simulink model "SD_Model"  (R2023b)
settings: Solver=FixedStepAuto  StartTime=1  StopTime=20  FixedStep=1  RelTol=1e-3
undefined symbols (not defined in the file): DiscIntNeverNeededParam
settings Model: Creator=eddyp  LastModifiedBy=eddyp

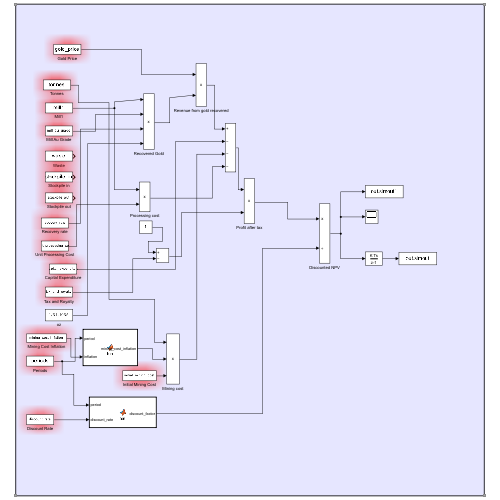
[thumbnail: Simulink's stored preview of the top-level diagram]
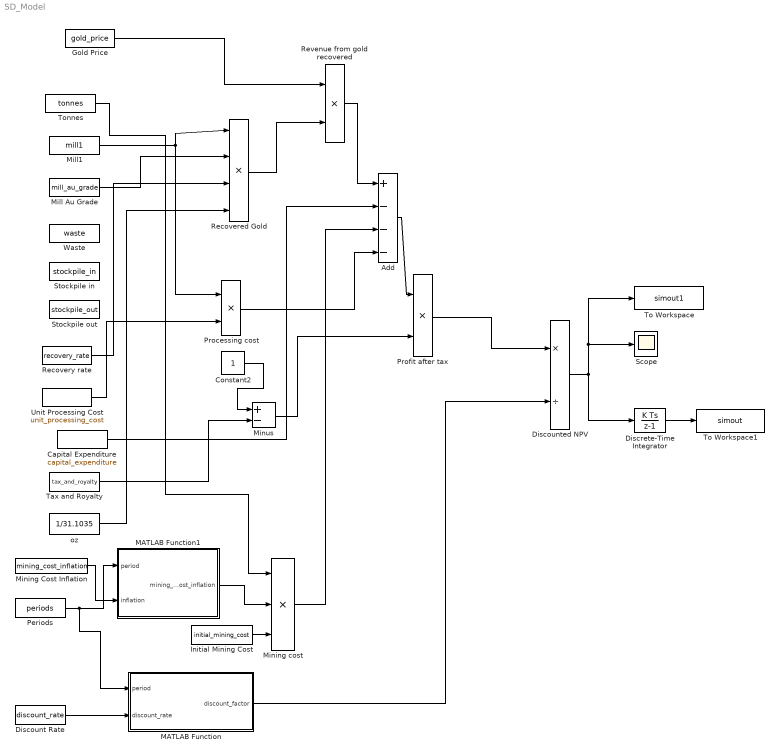
== system SD_Model ==
  Add : Sum  Inputs=+---
  Capital Expenditure : FromWorkspace  VariableName=capital_expenditure
  Constant2 : Constant
  Discount Rate : FromWorkspace  VariableName=discount_rate
  Discounted NPV : Product  Inputs=*/
  Discrete-Time Integrator : DiscreteIntegrator  SampleTime=-1  ICPrevOutput=DiscIntNeverNeededParam  ICPrevScaledInput=DiscIntNeverNeededParam
  Gold Price : FromWorkspace  VariableName=gold_price
  Initial Mining Cost : FromWorkspace  VariableName=initial_mining_cost
  MATLAB Function : MATLAB Function  TreatAsAtomicUnit=on
  MATLAB Function1 : MATLAB Function  TreatAsAtomicUnit=on
  Mill Au Grade : FromWorkspace  VariableName=mill_au_grade
  Mill1 : FromWorkspace  VariableName=mill1
  Mining Cost Inflation : FromWorkspace  VariableName=mining_cost_inflation
  Mining cost : Product  Inputs=3
  Minus : Sum  Inputs=+-
  Periods : FromWorkspace  VariableName=periods
  Processing cost : Product
  Profit after tax : Product
  Recovered Gold : Product  Inputs=4
  Recovery rate : FromWorkspace  VariableName=recovery_rate
  Revenue from gold recovered : Product
  Scope : Scope
  Stockpile in : FromWorkspace  VariableName=stockpile_in
  Stockpile out : FromWorkspace  VariableName=stockpile_out
  Tax and Royalty : FromWorkspace  VariableName=tax_and_royalty
  To Workspace : ToWorkspace  VariableName=simout1  SaveFormat=Timeseries  SampleTime=-1
  To Workspace1 : ToWorkspace  VariableName=simout  SaveFormat=Timeseries  SampleTime=-1
  Tonnes : FromWorkspace  VariableName=tonnes
  Unit Processing Cost : FromWorkspace  VariableName=unit_processing_cost
  Waste : FromWorkspace  VariableName=waste
  oz : Constant  Value=1/31.1035
  wires:
  Gold Price/1 -> Revenue from gold recovered/1
  Processing cost/1 -> Add/4
  Initial Mining Cost/1 -> Mining cost/3
  Profit after tax/1 -> Discounted NPV/1
  Mill Au Grade/1 -> Recovered Gold/2
  MATLAB Function/1(discount_factor) -> Discounted NPV/2
  Tax and Royalty/1 -> Minus/2
  Mill1/1 -> Recovered Gold/1, Processing cost/1
  Periods/1 -> MATLAB Function1/1(period), MATLAB Function/1(period)
  Constant2/1 -> Minus/1
  Minus/1 -> Profit after tax/2
  Mining cost/1 -> Add/3
  Tonnes/1 -> Mining cost/1
  Revenue from gold recovered/1 -> Add/1
  Capital Expenditure/1 -> Add/2
  Recovered Gold/1 -> Revenue from gold recovered/2
  Add/1 -> Profit after tax/1
  Unit Processing Cost/1 -> Processing cost/2
  Discounted NPV/1 -> Discrete-Time Integrator/1, To Workspace/1, Scope/1
  Recovery rate/1 -> Recovered Gold/3
  oz/1 -> Recovered Gold/4
  Discrete-Time Integrator/1 -> To Workspace1/1
  MATLAB Function1/1(mining_cost_inflation) -> Mining cost/2
  Discount Rate/1 -> MATLAB Function/2(discount_rate)
  Mining Cost Inflation/1 -> MATLAB Function1/2(inflation)

== matlab function SD_Model/MATLAB Function ==
  data: period input; discount_factor output; discount_rate input
function discount_factor = fcn(period, discount_rate)
    discount_factor = (1+(discount_rate/100))^(period-1);

== matlab function SD_Model/MATLAB Function1 ==
  data: period input; mining_cost_inflation output; inflation input
function mining_cost_inflation = fcn(period, inflation)
    mining_cost_inflation = (1+(inflation/100))^(period-1);
